simulink model "Subsystem"  (R2020a)
settings: Solver=VariableStepAuto  StartTime=0.0  StopTime=25  RelTol=1e-3
values from neighbouring files (symbols this model uses):
  I = 5.0    [ABSdd.sldd]
  Kf = 1.0    [ABSdd.sldd]
  PBmax = 1500.0    [ABSdd.sldd]
  Rr = 1.25    [ABSdd.sldd]
  TB = 0.01    [ABSdd.sldd]
  v0 = 88.0    [ABSdd.sldd]
settings Model: DataDictionary=ABSdd.sldd  Creator=HP  LastModifiedBy=HP
settings DataIOCC: SaveOutput=off  SaveTime=off

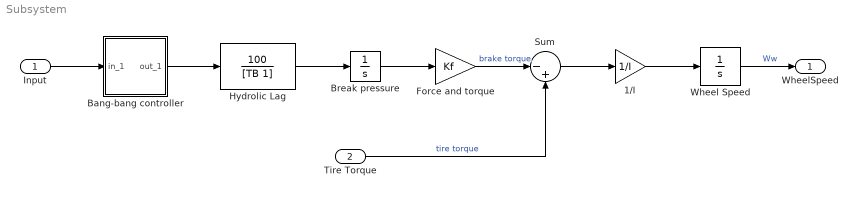
== system Subsystem ==
  Input : Inport  OutDataTypeStr=double  PortDimensions=1  SampleTime=0
  Tire Torque : Inport  Port=2  OutDataTypeStr=double  PortDimensions=1  SampleTime=0
  1/I : Gain  Gain=1/I  SaturateOnIntegerOverflow=on  OutDataTypeStr=Inherit: Same as input  ParamDataTypeStr=Inherit: Same as input
  Bang-bang controller : Subsystem
  Break pressure : Integrator  LimitOutput=on  UpperSaturationLimit=PBmax  LowerSaturationLimit=0
  Force and torque : Gain  Gain=Kf  SaturateOnIntegerOverflow=on  OutDataTypeStr=Inherit: Same as input  ParamDataTypeStr=Inherit: Same as input
  Hydrolic Lag : TransferFcn  Numerator=[100]  Denominator=[TB 1]
  Sum : Sum  Inputs=|-+
  Wheel Speed : Integrator  InitialCondition=v0/Rr  LimitOutput=on  UpperSaturationLimit=1000  LowerSaturationLimit=0
  WheelSpeed : Outport  OutDataTypeStr=double  PortDimensions=1  SampleTime=0  VectorParamsAs1DForOutWhenUnconnected=off
  wires:
  Break pressure/1 -> Force and torque/1
  Bang-bang controller/1(out_1) -> Hydrolic Lag/1
  Tire Torque/1 -> Sum/2  "tire torque"
  Wheel Speed/1 -> WheelSpeed/1  "Ww"
  Hydrolic Lag/1 -> Break pressure/1
  Force and torque/1 -> Sum/1  "brake torque"
  Input/1 -> Bang-bang controller/1(in_1)
  Sum/1 -> 1/I/1
  1/I/1 -> Wheel Speed/1

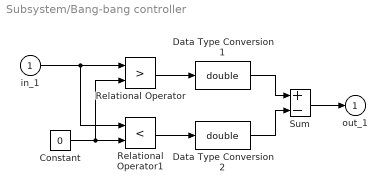
== system Subsystem/Bang-bang controller ==
  in_1 : Inport
  Constant : Constant  Value=0
  Data Type Conversion1 : DataTypeConversion  OutDataTypeStr=double  SaturateOnIntegerOverflow=on  RndMeth=Zero
  Data Type Conversion2 : DataTypeConversion  OutDataTypeStr=double  SaturateOnIntegerOverflow=on  RndMeth=Zero
  Relational Operator : RelationalOperator  Operator=>  OutDataTypeStr=boolean  RndMeth=Nearest  InputSameDT=on
  Relational Operator1 : RelationalOperator  Operator=<  OutDataTypeStr=boolean  RndMeth=Nearest  InputSameDT=on
  Sum : Sum  Inputs=+-  InputSameDT=on  SaturateOnIntegerOverflow=on  OutDataTypeStr=Inherit: Same as first input
  out_1 : Outport  InitialOutput=0  VectorParamsAs1DForOutWhenUnconnected=off
  wires:
  in_1/1 -> Relational Operator/1, Relational Operator1/1
  Constant/1 -> Relational Operator1/2, Relational Operator/2
  Relational Operator1/1 -> Data Type Conversion2/1
  Relational Operator/1 -> Data Type Conversion1/1
  Sum/1 -> out_1/1
  Data Type Conversion1/1 -> Sum/1
  Data Type Conversion2/1 -> Sum/2
